simulink model "preTrap60000"  (R2023a)
settings: Solver=FixedStepDiscrete  StartTime=0.0  StopTime=200  FixedStep=Ts  RelTol=1e-3
model workspace (MAT data in the model file):
  Ts = 0.002
  acoeff = 0.95
  amax = 0.1
  jcoeff = 0.1
  jmax = 1
  pf = 160
  reference_command = [0 0.002 0.004 0.006 0.008 0.01 0.012 0.014 0.016 0.018 0.02 0.022 ... (200002 elements, 100001x2)]
  v = 50
  vmax = 1.5
undefined symbols (not defined in the file or in its folder): sgn
settings Model: Creator=pietr  LastModifiedBy=giaco
settings SolverCC: AlgebraicLoopSolver=TrustRegion
settings DataIOCC: ExternalInput=az,alt,rot
settings DebuggingCC: UnconnectedInputMsg=warning  UnconnectedOutputMsg=warning  UnconnectedLineMsg=warning
settings ModelReferenceCC: EnableRefExpFcnMdlSchedulingChecks=on
settings RTWCC: DLArmComputeVersion=19.05

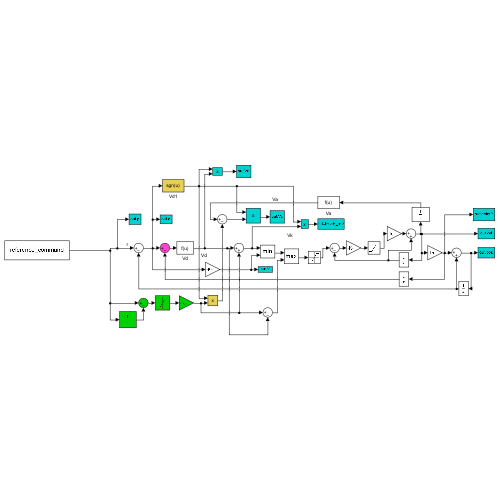
[thumbnail: Simulink's stored preview of the top-level diagram]
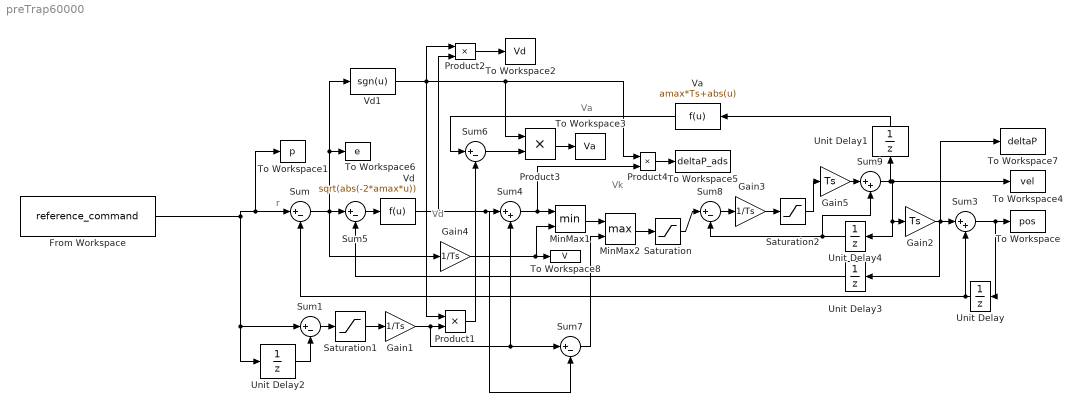
== system preTrap60000 ==
  note: Va
  note: Vd
  note: Vk
  note: r
  From Workspace : FromWorkspace  VariableName=reference_command
  Gain1 : Gain  Gain=1/Ts
  Gain2 : Gain  Gain=Ts
  Gain3 : Gain  Gain=1/Ts
  Gain4 : Gain  Gain=1/Ts
  Gain5 : Gain  Gain=Ts
  MinMax1 : MinMax  Inputs=2
  MinMax2 : MinMax  Function=max  Inputs=2
  Product{1..4} (4 alike) : Product
  Saturation : Saturate  UpperLimit=vmax  LowerLimit=-vmax
  Saturation1 : Saturate  UpperLimit=vmax*Ts  LowerLimit=-vmax*Ts
  Saturation2 : Saturate  UpperLimit=amax  LowerLimit=-amax
  Sum{,1,5..8} (6 alike) : Sum  Inputs=|+-
  Sum3 : Sum  Inputs=|++
  Sum4 : Sum  Inputs=|++
  Sum9 : Sum  Inputs=|++
  To Workspace : ToWorkspace  VariableName=pos  SampleTime=-1
  To Workspace1 : ToWorkspace  VariableName=p  SampleTime=-1
  To Workspace2 : ToWorkspace  VariableName=Vd  SampleTime=-1
  To Workspace3 : ToWorkspace  VariableName=Va  SampleTime=-1
  To Workspace4 : ToWorkspace  VariableName=vel  SampleTime=-1
  To Workspace5 : ToWorkspace  VariableName=deltaP_ads  SampleTime=-1
  To Workspace6 : ToWorkspace  VariableName=e  SampleTime=-1
  To Workspace7 : ToWorkspace  VariableName=deltaP  SampleTime=-1
  To Workspace8 : ToWorkspace  VariableName=V  SampleTime=-1
  Unit Delay{,1..4} (5 alike) : UnitDelay  SampleTime=-1  HasFrameUpgradeWarning=on
  Va : Fcn  Expr=amax*Ts+abs(u)
  Vd : Fcn  Expr=sqrt(abs(-2*amax*u))
  Vd1 : Fcn  Expr=sgn(u)
  wires:
  Sum/1 -> Sum5/1, Gain4/1, Vd1/1, To Workspace6/1
  Sum3/1 -> Unit Delay/1, To Workspace/1
  Va/1 -> Sum6/1
  Unit Delay/1 -> Sum/2, Sum3/2
  Sum6/1 -> Product3/2
  Gain2/1 -> To Workspace7/1, Sum3/1, Unit Delay3/1
  Unit Delay2/1 -> Sum1/2
  Saturation1/1 -> Gain1/1
  Sum1/1 -> Saturation1/1
  Unit Delay1/1 -> Va/1
  Product2/1 -> To Workspace2/1
  Product3/1 -> To Workspace3/1
  Product4/1 -> To Workspace5/1
  Product1/1 -> Sum6/2
  Sum5/1 -> Vd/1
  Sum9/1 -> To Workspace4/1, Unit Delay4/1, Gain2/1, Unit Delay1/1
  Sum4/1 -> Product4/2, MinMax1/1
  Unit Delay3/1 -> Sum5/2
  Vd1/1 -> Product2/1, Product1/1, Product4/1, Product3/1
  Gain4/1 -> MinMax1/2, To Workspace8/1
  Gain1/1 -> Sum7/1, Sum4/2, Product1/2
  Vd/1 -> Product2/2, Sum7/2, Sum4/1
  MinMax1/1 -> MinMax2/1
  Sum7/1 -> MinMax2/2
  MinMax2/1 -> Saturation/1
  From Workspace/1 -> Unit Delay2/1, Sum1/1, Sum/1, To Workspace1/1
  Saturation/1 -> Sum8/1
  Unit Delay4/1 -> Sum8/2, Sum9/2
  Sum8/1 -> Gain3/1
  Gain3/1 -> Saturation2/1
  Saturation2/1 -> Gain5/1
  Gain5/1 -> Sum9/1
